simulink model "sampleModel1401_3_sub_sub_sub"  (R2023a)
settings: Solver=VariableStepAuto  StartTime=0.0  StopTime=10.0  RelTol=1e-3
libraries: hdlsllib x1, simulink x1
settings Model: Creator=user1  LastModifiedBy=user1
settings OptimizationCC: BlockReduction=off  ConditionallyExecuteInputs=off

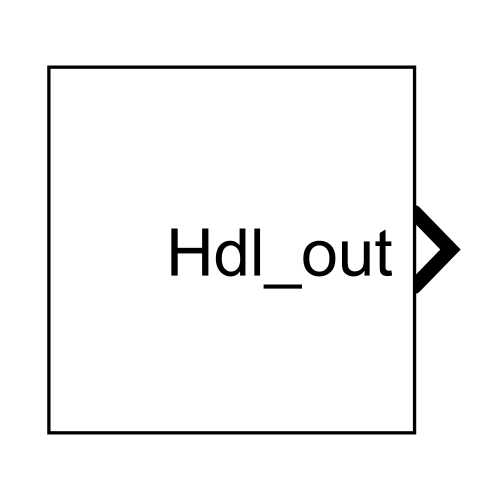
[thumbnail: Simulink's stored preview of the top-level diagram]
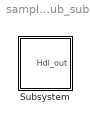
== system sampleModel1401_3_sub_sub_sub ==
  Subsystem : Subsystem

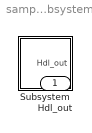
== system sampleModel1401_3_sub_sub_sub/Subsystem ==
  Subsystem : Subsystem
  Hdl_out : Outport  OutDataTypeStr=uint8

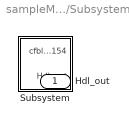
== system sampleModel1401_3_sub_sub_sub/Subsystem/Subsystem ==
  Subsystem : Subsystem
  Hdl_out : Outport  OutDataTypeStr=uint8

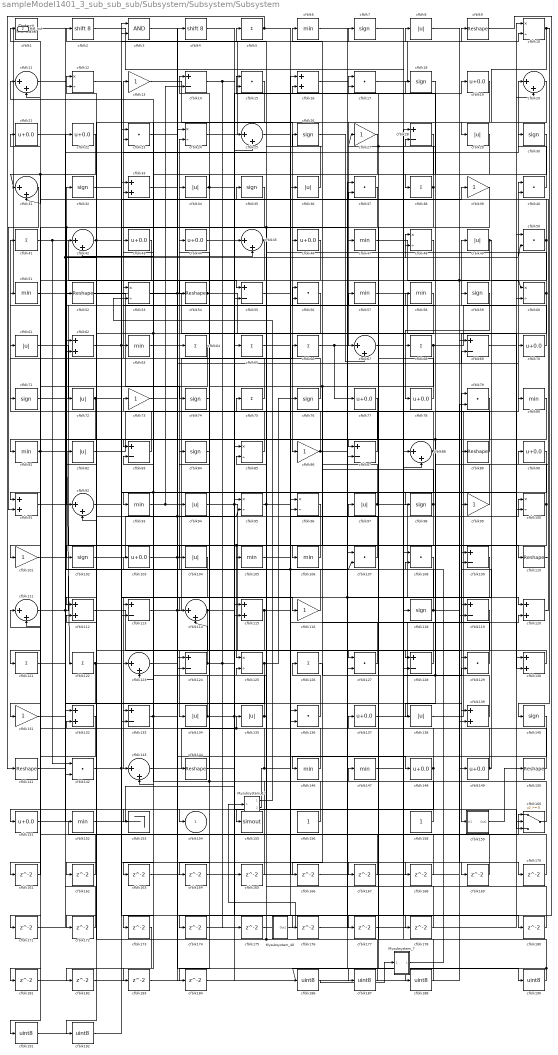
== system sampleModel1401_3_sub_sub_sub/Subsystem/Subsystem/Subsystem ==
  Mysubsystem_12 : Subsystem  TreatAsAtomicUnit=on  RTWFcnName=Mysubsystem_12
      settings: RTWFcnNameOpts=User specified  RTWFileNameOpts=Use function name
  Mysubsystem_40 : Subsystem  TreatAsAtomicUnit=on  RTWFcnName=Mysubsystem_40
      settings: RTWFcnNameOpts=User specified  RTWFileNameOpts=Use function name
  Mysubsystem_7 : Subsystem  TreatAsAtomicUnit=on  RTWFcnName=Mysubsystem_7
      settings: RTWFcnNameOpts=User specified  RTWFileNameOpts=Use function name
  cfblk1 : simulink/Logic and Bit Operations/Detect Increase  vinit=0.0  OutDataTypeStr=uint8
      settings: LibrarySourceBlock=|
      | hdlsllib/Logic and Bit
      | Operations/Detect
      | Increase
  cfblk{10,12,24,48,53,60,85,95..96,100,125} (11 alike) : Product  Inputs=*/  OutDataTypeStr=uint8  RndMeth=Zero  SaturateOnIntegerOverflow=on
  cfblk{13,27,39,73,86,99,101,116,131} (9 alike) : Gain  OutDataTypeStr=uint8
  cfblk{7,18,26,30,32,35,59,71,74,76,84,98,102,118,140} (15 alike) : Signum
  cfblk{19,21..22,43..44,46,70,77..78,90,103,137,148..149,151} (15 alike) : Bias  Bias=0.0  SaturateOnIntegerOverflow=off
  cfblk{8,29,34,36,49,61,72,82,94,97,104,134..135,138} (14 alike) : Abs  OutDataTypeStr=uint8  SaturateOnIntegerOverflow=off
  cfblk{6,47,51,57..58,63,80..81,93,105..106,146..147,152} (14 alike) : MinMax  OutDataTypeStr=uint8
  cfblk{15,17,23,37,40,50,56,79,107..108,127,129,136,142} (14 alike) : DotProduct  OutDataTypeStr=uint8
  cfblk{14,28,55,69,83,87,109,113,119,124,128,133} (12 alike) : Sum  Inputs=+-  OutDataTypeStr=uint8
  cfblk{11,20,25,31,42,45,67,88,92,111,114,123,143} (13 alike) : Sum  Inputs=|++  OutDataTypeStr=uint8
  cfblk{9,52,54,89,110,141,144,150} (8 alike) : Reshape
  cfblk{16,33,62,91,112,115,120,130,132,139} (10 alike) : Sum  OutDataTypeStr=uint8
  cfblk{5,38,41,64..66,68,75,121..122,126} (11 alike) : Sum  Inputs=+  OutDataTypeStr=uint8
  cfblk153 : Terminator
  cfblk155 : ToWorkspace  VariableName=simout  SaveFormat=Timeseries  SampleTime=-1
  cfblk156 : Constant  OutDataTypeStr=uint8  SampleTime=-1
  cfblk158 : Constant  OutDataTypeStr=uint8  SampleTime=-1
  cfblk159 : Subsystem
      settings: LibrarySourceBlock=|
      | hdlsllib/Ports &
      | Subsystems/Subsystem
  cfblk160 : Switch  OutDataTypeStr=uint8  SaturateOnIntegerOverflow=off  InputSameDT=off
  cfblk{161..178,180..184} (23 alike) : Delay  SampleTime=1
  cfblk{186..188,190..192} (6 alike) : DataTypeConversion  OutDataTypeStr=uint8  SaturateOnIntegerOverflow=off  RndMeth=Floor
  cfblk2 : ArithShift  BitShiftNumber=8
  cfblk3 : Logic  AllPortsSameDT=off  OutDataTypeStr=boolean
  cfblk4 : ArithShift  BitShiftNumber=8
  cfblk154 : Outport  OutDataTypeStr=uint8  VectorParamsAs1DForOutWhenUnconnected=off
  Hdl_out : Outport  Port=2  OutDataTypeStr=uint8
  wires:
  cfblk75/1 -> cfblk13/1
  cfblk96/1 -> cfblk123/2, cfblk125/1
  cfblk60/1 -> cfblk23/2, cfblk159/1(In1)
  cfblk19/1 -> cfblk67/1
  cfblk39/1 -> cfblk151/1
  cfblk26/1 -> cfblk67/2
  cfblk28/1 -> cfblk86/1
  cfblk41/1 -> cfblk55/1, cfblk142/1
  cfblk80/1 -> cfblk138/1, cfblk122/1
  cfblk125/1 -> cfblk162/1, cfblk76/1
  cfblk113/1 -> cfblk69/2, cfblk66/1
  cfblk59/1 -> cfblk78/1
  cfblk151/1 -> cfblk160/1
  cfblk22/1 -> cfblk31/2, cfblk31/1
  cfblk61/1 -> cfblk110/1
  cfblk24/1 -> cfblk7/1
  cfblk135/1 -> cfblk33/2, cfblk35/1
  cfblk72/1 -> cfblk161/1, cfblk10/2
  cfblk99/1 -> cfblk53/1
  cfblk36/1 -> cfblk2/1
  cfblk116/1 -> cfblk24/2
  cfblk114/1 -> cfblk58/1, cfblk134/1
  cfblk83/1 -> cfblk41/1
  cfblk110/1 -> cfblk40/1
  cfblk49/1 -> cfblk109/1, cfblk87/1
  cfblk140/1 -> cfblk146/1
  cfblk53/1 -> cfblk100/2, cfblk68/1
  cfblk104/1 -> cfblk143/1
  cfblk97/1 -> cfblk56/1, cfblk120/1
  cfblk70/1 -> cfblk49/1
  cfblk13/1 -> cfblk46/1
  cfblk136/1 -> cfblk126/1
  cfblk14/1 -> cfblk176/1, cfblk175/1
  cfblk2/1 -> cfblk118/1
  cfblk17/1 -> cfblk9/1
  cfblk118/1 -> cfblk170/1, cfblk32/1
  cfblk68/1 -> cfblk20/2, cfblk114/1, cfblk106/1
  cfblk52/1 -> cfblk74/1
  cfblk18/1 -> cfblk38/1
  cfblk77/1 -> cfblk143/2
  cfblk40/1 -> cfblk20/1
  cfblk10/1 -> cfblk29/1, cfblk140/1
  cfblk106/1 -> cfblk102/1
  cfblk7/1 -> cfblk88/1
  cfblk35/1 -> cfblk101/1, cfblk92/1
  cfblk159/1(Out1) -> cfblk150/1
  cfblk50/1 -> cfblk119/1, cfblk21/1
  cfblk95/1 -> cfblk75/1, cfblk36/1
  cfblk107/1 -> cfblk71/1
  cfblk30/1 -> cfblk93/1
  cfblk120/1 -> cfblk90/1
  cfblk94/1 -> cfblk59/1, cfblk127/1
  cfblk98/1 -> cfblk56/2, cfblk155/1
  cfblk91/1 -> cfblk52/1
  cfblk71/1 -> cfblk33/1
  cfblk89/1 -> cfblk28/2
  cfblk108/1 -> cfblk187/1
  cfblk137/1 -> cfblk79/1
  cfblk87/1 -> cfblk61/1
  cfblk152/1 -> cfblk115/1
  cfblk8/1 -> cfblk149/1
  cfblk45/1 -> cfblk55/2, cfblk5/1
  cfblk149/1 -> cfblk109/2, cfblk137/1
  cfblk79/1 -> cfblk87/2
  cfblk23/1 -> cfblk94/1
  cfblk29/1 -> cfblk154/1
  cfblk143/1 -> cfblk95/1
  cfblk66/1 -> cfblk77/1, cfblk119/2, cfblk160/2
  cfblk128/1 -> cfblk17/2, cfblk27/1
  cfblk3/1 -> cfblk190/1
  cfblk158/1 -> cfblk147/1
  cfblk78/1 -> cfblk15/1
  cfblk5/1 -> cfblk127/2, cfblk141/1
  cfblk134/1 -> cfblk42/2, cfblk168/1, cfblk65/1
  cfblk115/1 -> cfblk163/1, cfblk99/1, cfblk107/2
  cfblk56/1 -> cfblk172/1, cfblk83/1
  cfblk103/1 -> cfblk25/1, cfblk95/2, cfblk80/1
  cfblk139/1 -> cfblk6/1, cfblk18/1
  cfblk138/1 -> cfblk40/2
  cfblk11/1 -> cfblk72/1
  cfblk47/1 -> cfblk69/1, cfblk60/1
  cfblk69/1 -> cfblk130/1
  cfblk63/1 -> cfblk34/1
  cfblk105/1 -> cfblk100/1
  cfblk129/1 -> cfblk37/2
  cfblk57/1 -> cfblk130/2
  cfblk142/1 -> cfblk177/1, cfblk48/2, cfblk63/1
  cfblk156/1 -> cfblk44/1, cfblk43/1
  cfblk93/1 -> cfblk14/2, cfblk144/1
  cfblk85/1 -> cfblk73/1
  cfblk90/1 -> cfblk104/1
  cfblk130/1 -> cfblk123/1
  cfblk15/1 -> cfblk113/1
  cfblk62/1 -> cfblk116/1
  cfblk76/1 -> cfblk51/1
  cfblk112/1 -> cfblk129/1
  cfblk127/1 -> cfblk26/1
  cfblk4/1 -> cfblk160/3
  cfblk102/1 -> cfblk45/1
  cfblk109/1 -> cfblk113/2
  cfblk33/1 -> cfblk8/1
  cfblk25/1 -> cfblk19/1
  cfblk54/1 -> Hdl_out/1, cfblk136/1
  cfblk100/1 -> cfblk15/2, cfblk124/2
  cfblk81/1 -> cfblk57/1, cfblk121/1
  cfblk101/1 -> cfblk45/2
  cfblk1/1 -> cfblk89/1
  cfblk34/1 -> cfblk14/1, cfblk128/1
  cfblk111/1 -> cfblk30/1, cfblk16/1
  cfblk42/1 -> cfblk54/1, cfblk12/1
  cfblk82/1 -> cfblk50/1
  cfblk51/1 -> cfblk131/1
  cfblk84/1 -> cfblk64/1
  cfblk150/1 -> cfblk132/2
  cfblk131/1 -> cfblk152/1
  cfblk38/1 -> cfblk17/1, cfblk133/1, cfblk105/1
  cfblk121/1 -> cfblk50/2, cfblk22/1
  cfblk122/1 -> cfblk142/2, cfblk39/1
  cfblk73/1 -> cfblk96/2
  cfblk144/1 -> cfblk25/2
  cfblk37/1 -> cfblk81/1
  cfblk86/1 -> cfblk70/1, cfblk62/2
  cfblk160/1 -> cfblk84/1
  cfblk43/1 -> cfblk91/1
  cfblk31/1 -> cfblk91/2
  cfblk124/1 -> cfblk114/2, cfblk165/1, cfblk48/1
  cfblk6/1 -> cfblk128/2
  cfblk146/1 -> cfblk135/1, cfblk111/2
  cfblk21/1 -> cfblk139/1
  cfblk92/1 -> cfblk98/1
  cfblk88/1 -> cfblk11/2, cfblk133/2, cfblk153/1
  cfblk48/1 -> cfblk136/2
  cfblk20/1 -> cfblk112/1
  cfblk44/1 -> cfblk16/2
  cfblk148/1 -> cfblk184/1, cfblk92/2
  cfblk123/1 -> cfblk4/1
  cfblk133/1 -> cfblk83/2, cfblk148/1
  cfblk141/1 -> cfblk103/1
  cfblk12/1 -> cfblk47/1
  cfblk147/1 -> cfblk129/2
  cfblk161/1 -> cfblk1/1
  cfblk162/1 -> cfblk111/1
  cfblk163/1 -> cfblk96/1
  cfblk74/1 -> cfblk164/1
  cfblk164/1 -> cfblk88/2
  cfblk165/1 -> cfblk11/1
  cfblk126/1 -> cfblk166/1
  cfblk166/1 -> cfblk139/2
  cfblk65/1 -> cfblk167/1
  cfblk167/1 -> cfblk85/1
  cfblk168/1 -> cfblk112/2
  cfblk32/1 -> cfblk169/1
  cfblk169/1 -> cfblk124/1
  cfblk170/1 -> cfblk42/1
  cfblk46/1 -> cfblk171/1
  cfblk171/1 -> cfblk62/1
  cfblk172/1 -> cfblk132/1
  cfblk27/1 -> cfblk173/1
  cfblk9/1 -> cfblk174/1
  cfblk174/1 -> cfblk37/1
  cfblk175/1 -> cfblk28/1
  cfblk176/1 -> cfblk60/2
  cfblk177/1 -> cfblk10/1
  cfblk55/1 -> cfblk178/1
  cfblk178/1 -> cfblk125/2
  cfblk67/1 -> cfblk180/1
  cfblk180/1 -> cfblk107/1
  cfblk64/1 -> cfblk181/1
  cfblk181/1 -> cfblk23/1
  cfblk119/1 -> cfblk182/1
  cfblk182/1 -> cfblk79/2
  cfblk58/1 -> cfblk183/1
  cfblk183/1 -> cfblk24/1
  cfblk184/1 -> cfblk115/2
  cfblk187/1 -> cfblk85/2, cfblk12/2
  cfblk16/1 -> cfblk188/1
  cfblk188/1 -> cfblk108/1
  cfblk190/1 -> cfblk97/1, cfblk186/1
  cfblk132/1 -> cfblk191/1
  cfblk191/1 -> cfblk3/1
  cfblk173/1 -> cfblk192/1
  cfblk192/1 -> cfblk3/2
  cfblk186/1 -> Mysubsystem_7/1(In1)
  Mysubsystem_7/1(Out1) -> cfblk108/2
  Mysubsystem_12/2(Out2) -> cfblk120/2, cfblk82/1
  Mysubsystem_12/1(Out1) -> cfblk53/2
  Mysubsystem_40/1(Out1) -> Mysubsystem_12/1(In1)

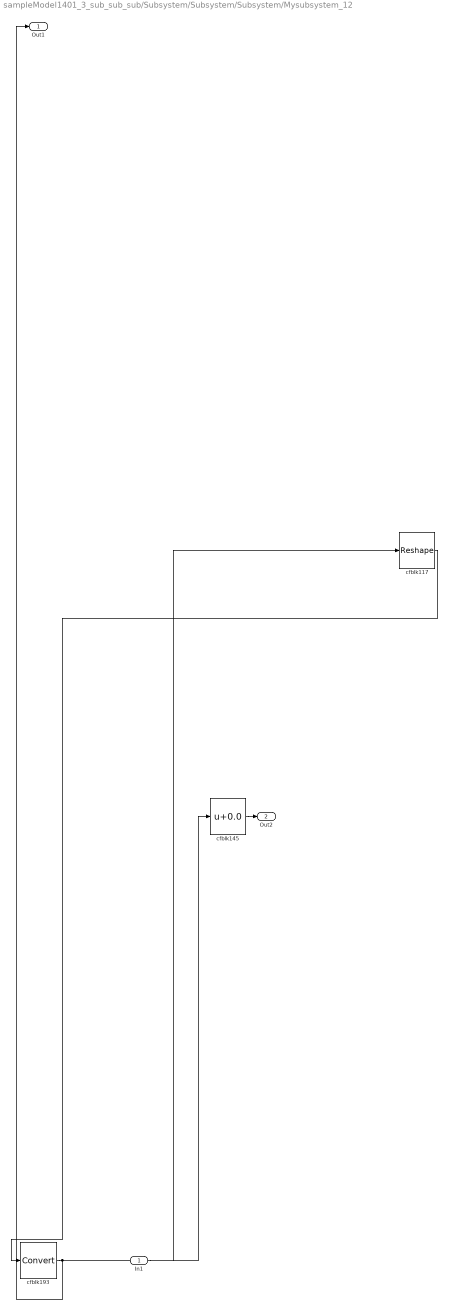
== system sampleModel1401_3_sub_sub_sub/Subsystem/Subsystem/Subsystem/Mysubsystem_12 ==
  In1 : Inport
  cfblk117 : Reshape
  cfblk145 : Bias  Bias=0.0  SaturateOnIntegerOverflow=off
  cfblk193 : DataTypeConversion  SaturateOnIntegerOverflow=off  RndMeth=Floor
  Out1 : Outport
  Out2 : Outport  Port=2
  wires:
  In1/1 -> cfblk117/1
  cfblk145/1 -> Out2/1
  cfblk193/1 -> cfblk145/1, Out1/1
  cfblk117/1 -> cfblk193/1

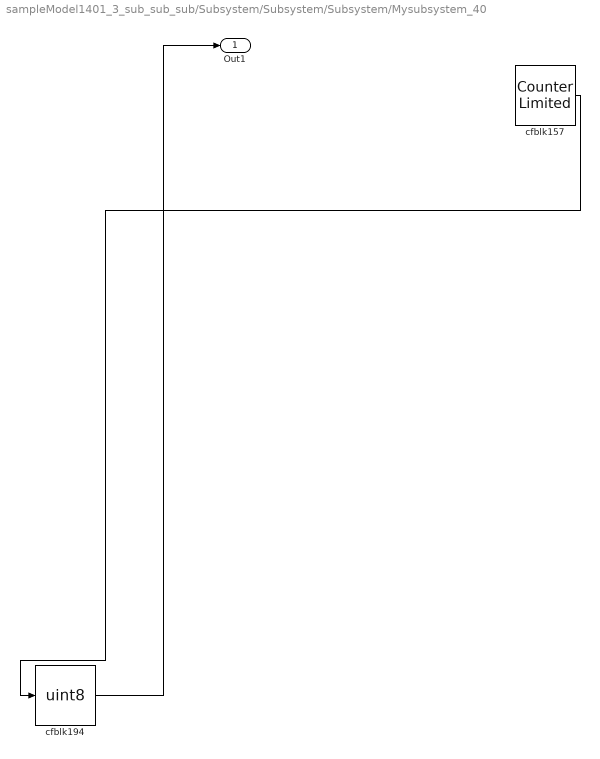
== system sampleModel1401_3_sub_sub_sub/Subsystem/Subsystem/Subsystem/Mysubsystem_40 ==
  cfblk157 : hdlsllib/Sources/Counter Limited  uplimit=7  tsamp=-1
  cfblk194 : DataTypeConversion  OutDataTypeStr=uint8  SaturateOnIntegerOverflow=off  RndMeth=Floor
  Out1 : Outport
  wires:
  cfblk194/1 -> Out1/1
  cfblk157/1 -> cfblk194/1

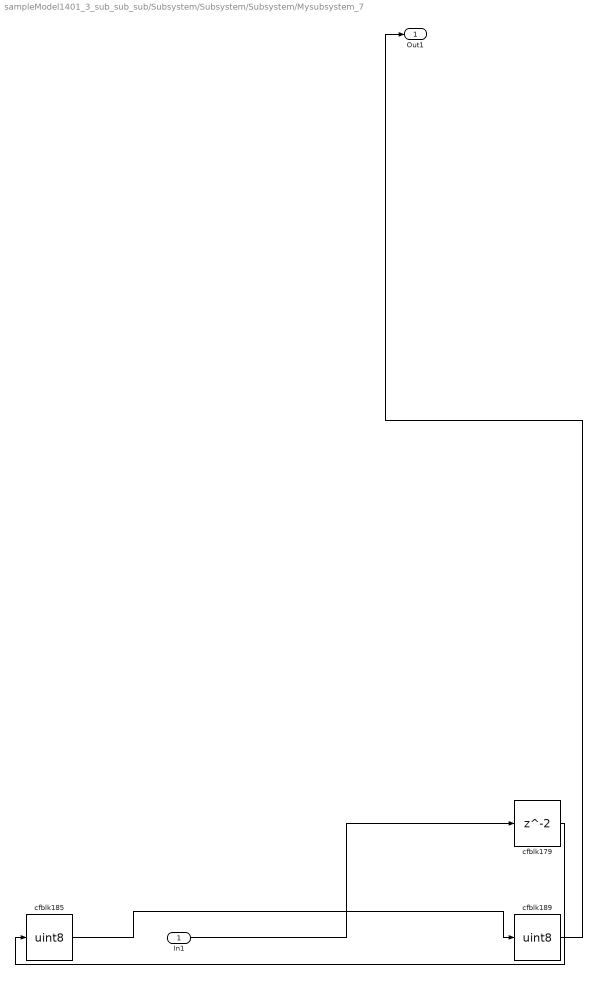
== system sampleModel1401_3_sub_sub_sub/Subsystem/Subsystem/Subsystem/Mysubsystem_7 ==
  In1 : Inport
  cfblk179 : Delay  SampleTime=1
  cfblk185 : DataTypeConversion  OutDataTypeStr=uint8  SaturateOnIntegerOverflow=off  RndMeth=Floor
  cfblk189 : DataTypeConversion  OutDataTypeStr=uint8  SaturateOnIntegerOverflow=off  RndMeth=Floor
  Out1 : Outport
  wires:
  cfblk189/1 -> Out1/1
  In1/1 -> cfblk179/1
  cfblk185/1 -> cfblk189/1
  cfblk179/1 -> cfblk185/1

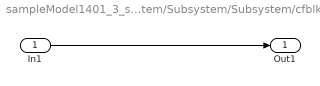
== system sampleModel1401_3_sub_sub_sub/Subsystem/Subsystem/Subsystem/cfblk159 ==
  In1 : Inport
  Out1 : Outport
  wires:
  In1/1 -> Out1/1
